simulink model "controller_TRIAD_minimal"  (R2016b)
settings: Solver=VariableStepAuto  StartTime=0.0  StopTime=200  RelTol=1e-3
values from neighbouring files (symbols this model uses):
  quat_cmd = quat_cmd/norm(quat_cmd)    [ctrl_TRIAD_test.m]
  var_mult_mt = 10000    [ctrl_TRIAD_test.m]
  var_mult_sun = 10000    [ctrl_TRIAD_test.m]
undefined symbols (not defined in the file or in its folder): sim_params
libraries: dynamics_lib x2, pd_control_lib x1, triad_coarse_estimator x1
settings Model: Creator=sexymathemagician  LastModifiedBy=sexymathemagician

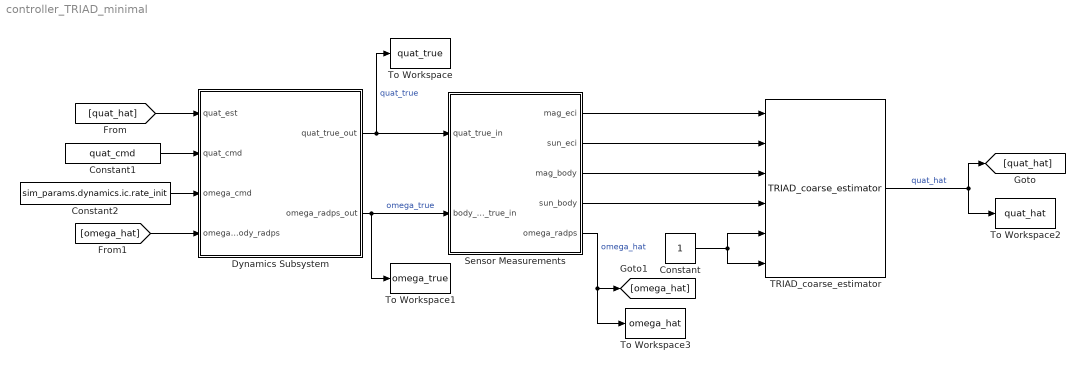
== system controller_TRIAD_minimal ==
  Constant : Constant
  Constant1 : Constant  Value=quat_cmd
  Constant2 : Constant  Value=sim_params.dynamics.ic.rate_init
  Dynamics Subsystem : Subsystem
  "Sensor Measurements " : Subsystem
  TRIAD_coarse_estimator : triad_coarse_estimator/TRIAD_coarse_estimator
  To Workspace : ToWorkspace  VariableName=quat_true  SaveFormat=Timeseries  SampleTime=-1
  To Workspace1 : ToWorkspace  VariableName=omega_true  SaveFormat=Timeseries  SampleTime=-1
  To Workspace2 : ToWorkspace  VariableName=quat_hat  SaveFormat=Timeseries  SampleTime=-1
  To Workspace3 : ToWorkspace  VariableName=omega_hat  SaveFormat=Timeseries  SampleTime=-1
  wires:
  "Sensor Measurements "/1(mag_eci) -> TRIAD_coarse_estimator/1
  "Sensor Measurements "/2(sun_eci) -> TRIAD_coarse_estimator/2
  "Sensor Measurements "/3(mag_body) -> TRIAD_coarse_estimator/3
  "Sensor Measurements "/4(sun_body) -> TRIAD_coarse_estimator/4
  Dynamics Subsystem/1(quat_true_out) -> "Sensor Measurements "/1(quat_true_in), To Workspace/1  "quat_true"
  Dynamics Subsystem/2(omega_radps_out) -> "Sensor Measurements "/2(body_rates_true_in), To Workspace1/1  "omega_true"
  [quat_hat] -> Dynamics Subsystem/1(quat_est)
  "Sensor Measurements "/5(omega_radps) -> To Workspace3/1, [omega_hat]  "omega_hat"
  [omega_hat] -> Dynamics Subsystem/4(omega_body_radps)
  Constant1/1 -> Dynamics Subsystem/2(quat_cmd)
  Constant2/1 -> Dynamics Subsystem/3("omega_cmd ")
  Constant/1 -> TRIAD_coarse_estimator/6, TRIAD_coarse_estimator/5
  TRIAD_coarse_estimator/1 -> To Workspace2/1, [quat_hat]  "quat_hat"

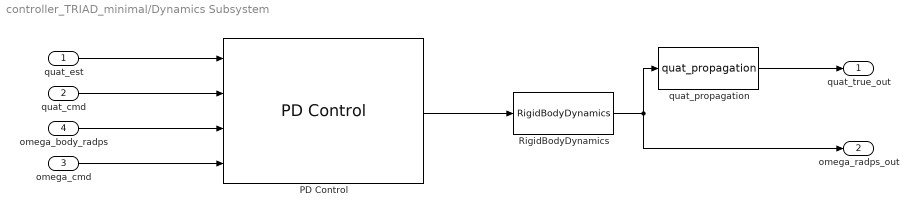
== system controller_TRIAD_minimal/Dynamics Subsystem ==
  quat_est : Inport
  quat_cmd : Inport  Port=2
  "omega_cmd " : Inport  Port=3
  omega_body_radps : Inport  Port=4
  PD Control : pd_control_lib/PD Control
  RigidBodyDynamics : dynamics_lib/Dynamics/RigidBodyDynamics
  quat_propagation : dynamics_lib/Dynamics/quat_propagation
  quat_true_out : Outport
  omega_radps_out : Outport  Port=2
  wires:
  "omega_cmd "/1 -> PD Control/4
  quat_est/1 -> PD Control/1
  quat_cmd/1 -> PD Control/2
  omega_body_radps/1 -> PD Control/3
  RigidBodyDynamics/1 -> omega_radps_out/1, quat_propagation/1
  quat_propagation/1 -> quat_true_out/1
  PD Control/1 -> RigidBodyDynamics/1

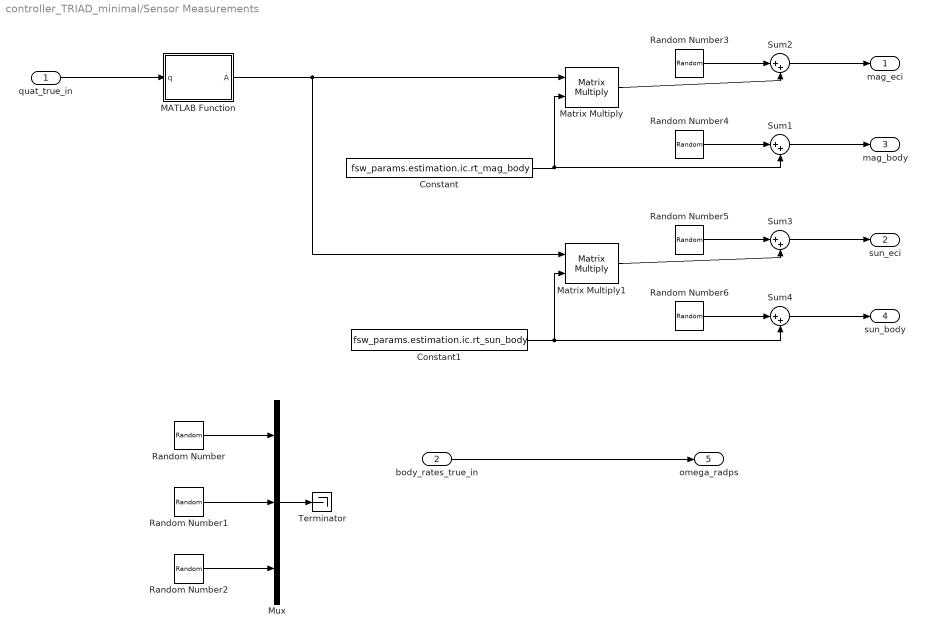
== system controller_TRIAD_minimal/Sensor Measurements  ==
  quat_true_in : Inport
  body_rates_true_in : Inport  Port=2
  Constant : Constant  Value=fsw_params.estimation.ic.rt_mag_body
  Constant1 : Constant  Value=fsw_params.estimation.ic.rt_sun_body
  MATLAB Function : MATLAB Function  TreatAsAtomicUnit=on
  Matrix Multiply : Product  Multiplication=Matrix(*)
  Matrix Multiply1 : Product  Multiplication=Matrix(*)
  Mux : Mux  Inputs=3
  Random Number : RandomNumber  Variance=(sim_params.sensors.gyro.arw)^2/(60*60)  SampleTime=0.1
  Random Number1 : RandomNumber  Variance=(sim_params.sensors.gyro.arw)^2/(60*60)  SampleTime=0.1
  Random Number2 : RandomNumber  Variance=(sim_params.sensors.gyro.arw)^2/(60*60)  SampleTime=0.1
  Random Number3 : RandomNumber  Variance=var_mult_mt*(sim_params.sensors.magnetometer.deg_err)^2/(60*60)  SampleTime=0.1
  Random Number4 : RandomNumber  Variance=var_mult_mt*(sim_params.sensors.magnetometer.deg_err)^2/(60*60)  SampleTime=0.1
  Random Number5 : RandomNumber  Variance=var_mult_sun*(sim_params.sensors.sun_sensor.deg_err)^2/(60*60)  SampleTime=0.1
  Random Number6 : RandomNumber  Variance=var_mult_mt*(sim_params.sensors.sun_sensor.deg_err)^2/(60*60)  SampleTime=0.1
  Sum{1..4} (4 alike) : Sum  Inputs=|++
  Terminator : Terminator
  mag_eci : Outport
  sun_eci : Outport  Port=2
  mag_body : Outport  Port=3
  sun_body : Outport  Port=4
  omega_radps : Outport  Port=5
  wires:
  quat_true_in/1 -> MATLAB Function/1(q)
  Constant/1 -> Sum1/2, Matrix Multiply/2
  Constant1/1 -> Sum4/2, Matrix Multiply1/2
  Random Number/1 -> Mux/1
  Random Number1/1 -> Mux/2
  Random Number2/1 -> Mux/3
  body_rates_true_in/1 -> omega_radps/1
  Mux/1 -> Terminator/1
  MATLAB Function/1(A) -> Matrix Multiply1/1, Matrix Multiply/1
  Random Number3/1 -> Sum2/1
  Matrix Multiply/1 -> Sum2/2
  Sum2/1 -> mag_eci/1
  Random Number4/1 -> Sum1/1
  Sum1/1 -> mag_body/1
  Random Number5/1 -> Sum3/1
  Random Number6/1 -> Sum4/1
  Sum3/1 -> sun_eci/1
  Sum4/1 -> sun_body/1
  Matrix Multiply1/1 -> Sum3/2

== matlab function controller_TRIAD_minimal/Sensor Measurements /MATLAB Function ==
  data: q input; A output
function A = quatToMatrix(q)
%#codegen

eta = q(1);
eps = q(2:4);

A = (2*eta^2 -1)*eye(3) + 2*(eps*eps') - 2*eta*skew(eps);


end

function cross = skew(a)
%#codegen

cross = [0 -a(3) a(2);
         a(3) 0 -a(1);
        -a(2) a(1) 0];

end
